simulink model "SOE"  (R2021a)
settings: Solver=VariableStepAuto  StartTime=0.0  StopTime=10.0  RelTol=1e-3
settings Model: Creator=SAHIL  LastModifiedBy=SAHIL

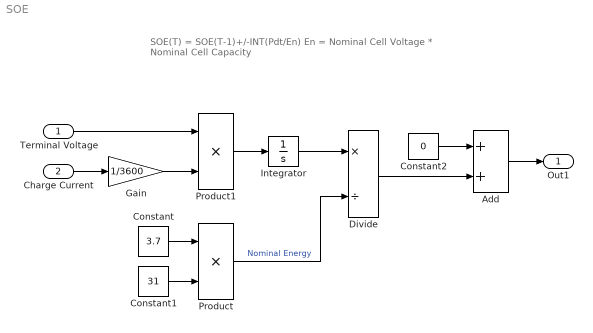
== system SOE ==
  note: SOE(T) = SOE(T-1)+/-INT(Pdt/En)
      |
      | En = Nominal Cell Voltage * Nominal Cell Capacity
  Terminal Voltage : Inport
  Charge Current : Inport  Port=2
  Add : Sum
  Constant : Constant  Value=3.7
  Constant1 : Constant  Value=31
  Constant2 : Constant  Value=0
  Divide : Product  Inputs=*/
  Gain : Gain  Gain=1/3600
  Integrator : Integrator
  Product : Product
  Product1 : Product
  Out1 : Outport
  wires:
  Add/1 -> Out1/1
  Charge Current/1 -> Gain/1
  Constant2/1 -> Add/1
  Terminal Voltage/1 -> Product1/1
  Divide/1 -> Add/2
  Product1/1 -> Integrator/1
  Integrator/1 -> Divide/1
  Constant1/1 -> Product/2
  Product/1 -> Divide/2  "Nominal Energy"
  Gain/1 -> Product1/2
  Constant/1 -> Product/1
